simulink model "Chromatic Conveyor"  (R2025a)
settings: Solver=ode3  StartTime=0.0  StopTime=10  RelTol=1e-3  EnableMultiTasking=on
libraries: legoev3lib x4
settings Model: FPTRunName=Active  ExtModeTrigDuration=2  Creator=tstaib  LastModifiedBy=tstaib
settings SolverCC: AlgebraicLoopSolver=TrustRegion  PositivePriorityOrder=on
settings DataIOCC: LimitDataPoints=on  SaveFormat=Array
settings OptimizationCC: ExpressionDepthLimit=2147483647.0  LifeSpan=Inf  MaxStackSize=64
settings DebuggingCC: UnderspecifiedInitializationDetection=Classic  MergeDetectMultiDrivingBlocksExec=none  FcnCallInpInsideContextMsg=warning  UnconnectedInputMsg=warning  UnconnectedOutputMsg=warning  UnconnectedLineMsg=warning  AllowSymbolicDim=off  StateNameClashWarn=warning  SFUnexpectedBacktrackingDiag=warning  SFNoUnconditionalDefaultTransitionDiag=warning  SFExecutionAtInitializationDiag=none  ArithmeticOperatorsInVariantConditions=warning
settings HardwareCC: ProdBitPerPointer=32.0  ProdBitPerSizeT=32.0  ProdBitPerPtrDiffT=32.0  ProdLargestAtomicInteger=Long  ProdWordSize=32.0  ProdHWDeviceType=ARM Compatible->ARM 9  UseEmbeddedCoderFeatures=off
settings ModelReferenceCC: EnableRefExpFcnMdlSchedulingChecks=on  PropagateSignalLabelsOutOfModel=off
settings SFSimCC: SimUseLocalCustomCode=off  CustomCodeUndefinedFunction=UseInterfaceOnly
settings RTWCC: SystemTargetFile=ert.tlc  HardwareBoard=LEGO MINDSTORMS EV3  TemplateMakefile=ert_default_tmf  GenerateReport=on  RTWVerbose=off  RTWUseLocalCustomCode=off  Toolchain=Sourcery G++ Lite v2009q3  BuildConfiguration=Faster Runs  LaunchReport=on  GPUComputeCapability=3.5  Description=Embedded Coder
settings CodeAppCC: ForceParamTrailComments=on  OperatorAnnotations=on  StateflowObjectComments=on  MATLABSourceComments=on
settings ERTTargetCC: ExtModeTransport=0.0  ExtModeStaticAlloc=off  ExtModeMexFile=ext_comm  ExtModeIntrfLevel=Level1  InlinedParameterPlacement=Hierarchical  DynamicArrayContainerType=coder::array  MultiwordLength=2048.0  ERTCustomFileBanners=off  SupportContinuousTime=on  SupportNonInlinedSFcns=on  RemoveResetFunc=off  SupportVariableSizeSignals=on  ModelStepFunctionPrototypeControlCompliant=off
settings ConfigComp: CovMetricSettings=dw  CovSaveCumulativeToWorkspaceVar=on  CovSaveSingleToWorkspaceVar=on  CovExternalEMLEnable=off  CovSFcnEnable=off

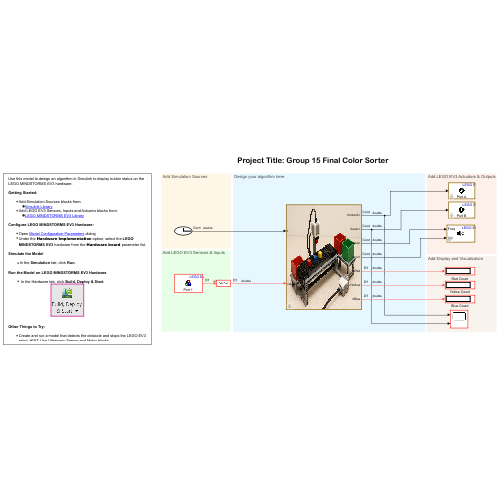
[thumbnail: Simulink's stored preview of the top-level diagram]
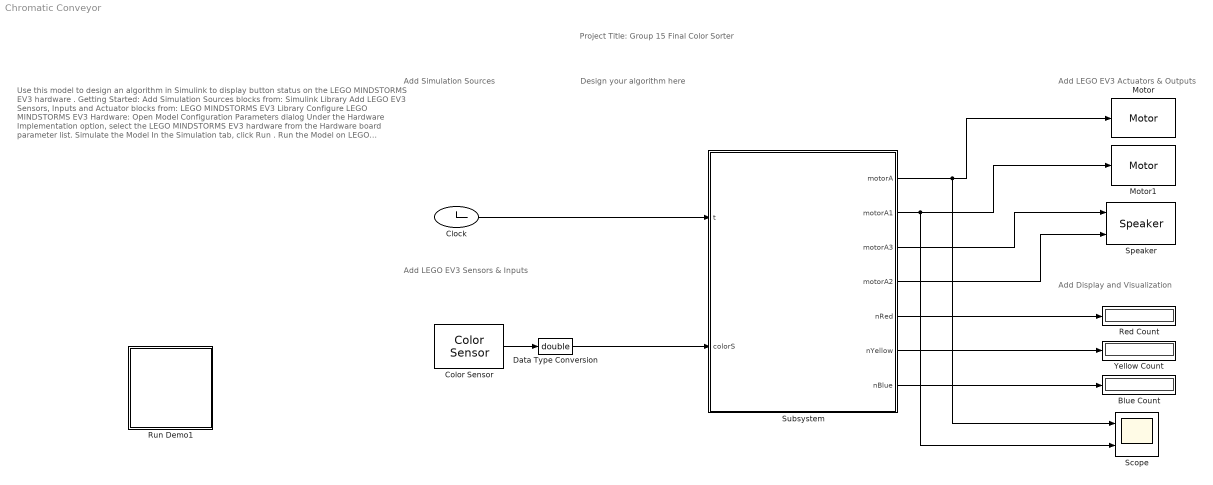
== system Chromatic Conveyor ==
  note: Project Title: Group 15 Final Color Sorter
  note: Add LEGO EV3 Sensors & Inputs
  note: Add LEGO EV3 Actuators & Outputs
  note: Add Display and Visualization
  note: Design your algorithm here
  note: Add Simulation Sources
  note: Use this model to design an algorithm in Simulink to display button status on the LEGO MINDSTORMS EV3 hardware .
      |
      | Getting Started:
      |
      | Add Simulation Sources blocks from:
      | Simulink Library
      | Add LEGO EV3 Sensors, Inputs and Actuator blocks from:
      | LEGO MINDSTORMS EV3 Library
      |
      | Configure LEGO MINDSTORMS EV3 Hardware:
      |
      | Open Model Configuration Parameters dialog
      | Under the Hardware Implementation option, select the LEGO MINDSTORMS EV3 hardware from the Hardware board parameter list.
      |
      | Simulate the Model
      |
      | In the Simulation tab, click Run .
      |
      | Run the Model on LEGO MINDSTORMS EV3 Hardware
      |
      | In the Hardware tab, click Build, Deploy & Start .
      |
      | Other Things to Try:
      |
      | Create and run a model that detects the obstacle and stops the LEGO EV3 robot. HINT: Use Ultrasonic Sensor and Motor blocks.
  Blue Count : Display
  Clock : Clock
  Color Sensor : legoev3lib/Color Sensor  portNumber=1  mode=Reflected light intensity  sampleTime=0.5
  Data Type Conversion : DataTypeConversion  OutDataTypeStr=double  SaturateOnIntegerOverflow=off  RndMeth=Floor
  Motor : legoev3lib/Motor  sportNumber=A  sstopAction=Brake
  Motor1 : legoev3lib/Motor  sportNumber=B  sstopAction=Brake
  Red Count : Display
  Run Demo1 : Subsystem  Description=Controls host-side RTDX processing.
      mask Display: pic=imread('ev3BuildDeployandStart.png');image(pic);
  Scope : Scope  NumInputPorts=2
  Speaker : legoev3lib/Speaker  sinputMode=Frequency and volume  sspeakerFreq=100  sspeakerVolume=50  sspeakerDuration=100
  Subsystem : Subsystem  mask{stopTime=120, speed=30, redR=[70 95], yellowR=[96 100], blueR=[12 20]}
      mask prompts: stopTime "Time On (sec)"; speed "Conveyor Speed"; redR "Red Range [min max]"; yellowR "Yellow Range [min max]"; blueR "Blue Range [min max]"
      mask Display: image('image.png');
  Yellow Count : Display
  wires:
  Clock/1 -> Subsystem/1(t)
  Color Sensor/1 -> Data Type Conversion/1
  Subsystem/1(motorA) -> Scope/1, Motor/1
  Subsystem/2(motorA1) -> Scope/2, Motor1/1
  Data Type Conversion/1 -> Subsystem/2(colorS)
  Subsystem/3(motorA3) -> Speaker/1
  Subsystem/4(motorA2) -> Speaker/2
  Subsystem/5(nRed) -> Red Count/1
  Subsystem/6(nYellow) -> Yellow Count/1
  Subsystem/7(nBlue) -> Blue Count/1

== system Chromatic Conveyor/Run Demo1 ==

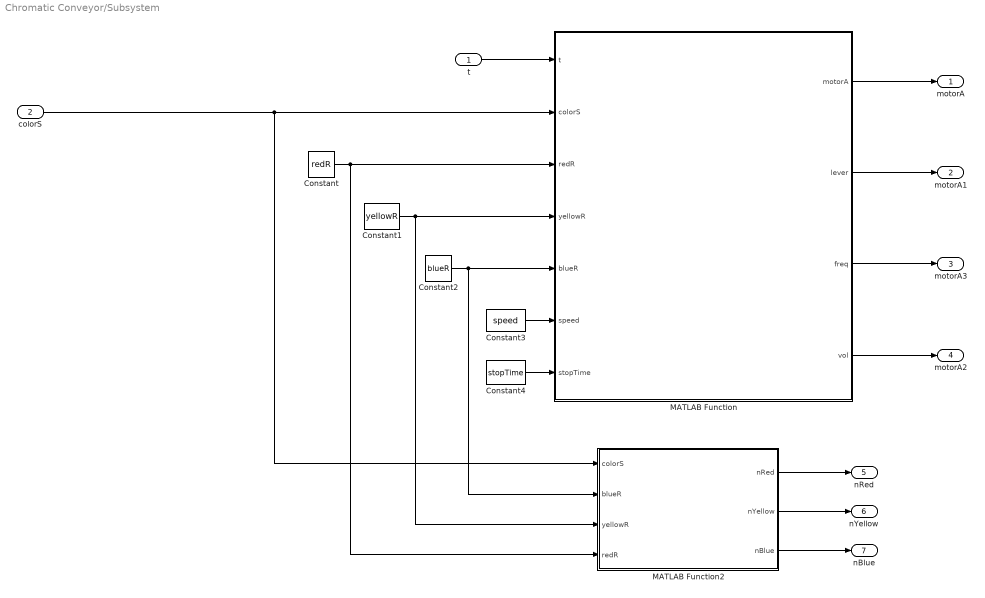
== system Chromatic Conveyor/Subsystem ==
  t : Inport
  colorS : Inport  Port=2
  Constant : Constant  Value=redR
  Constant1 : Constant  Value=yellowR
  Constant2 : Constant  Value=blueR
  Constant3 : Constant  Value=speed
  Constant4 : Constant  Value=stopTime
  MATLAB Function : MATLAB Function  TreatAsAtomicUnit=on
  MATLAB Function2 : MATLAB Function  TreatAsAtomicUnit=on
  motorA : Outport
  motorA1 : Outport  Port=2
  motorA3 : Outport  Port=3
  motorA2 : Outport  Port=4
  nRed : Outport  Port=5
  nYellow : Outport  Port=6
  nBlue : Outport  Port=7
  wires:
  Constant4/1 -> MATLAB Function/7(stopTime)
  Constant3/1 -> MATLAB Function/6(speed)
  Constant2/1 -> MATLAB Function2/2(blueR), MATLAB Function/5(blueR)
  Constant1/1 -> MATLAB Function2/3(yellowR), MATLAB Function/4(yellowR)
  Constant/1 -> MATLAB Function2/4(redR), MATLAB Function/3(redR)
  t/1 -> MATLAB Function/1(t)
  MATLAB Function/1(motorA) -> motorA/1
  MATLAB Function/2(lever) -> motorA1/1
  MATLAB Function/4(vol) -> motorA2/1
  MATLAB Function/3(freq) -> motorA3/1
  MATLAB Function2/1(nRed) -> nRed/1
  MATLAB Function2/2(nYellow) -> nYellow/1
  MATLAB Function2/3(nBlue) -> nBlue/1
  colorS/1 -> MATLAB Function2/1(colorS), MATLAB Function/2(colorS)

== matlab function Chromatic Conveyor/Subsystem/MATLAB Function ==
  data: t input; motorA output; lever output; freq output; colorS input; redR input; yellowR input; blueR input; vol output; speed input; stopTime input
function [motorA, lever, freq, vol] = fcn(t, colorS, redR, yellowR, blueR, speed, stopTime)

% defaults
motorA = 0;
lever  = 0;
vol    = 0;
freq   = 0;

% persistent state for per-brick timing
% state: 0 = idle, 1 = red, 2 = yellow, 3 = blue
persistent state startTime

if isempty(state)
    state     = 0;
    startTime = 0;
end

% 
if t >= stopTime
    state     = 0;     % reset state
    motorA    = 0;
    lever     = 0;
    vol       = 0;
    freq      = 0;
    return;
end

% Conveyor Run time for each brick
runTime = 4;   % seconds


% If we are idle, check the sensor and possibly start a
% new sorting cycle for the current brick.
if state == 0
    if colorS >= redR(1) && colorS <= redR(2)
        state     = 1;      % RED
        startTime = t;
    elseif colorS >= yellowR(1) && colorS <= yellowR(2)
        state     = 2;      % YELLOW
        startTime = t;
    elseif colorS >= blueR(1) && colorS <= blueR(2)
        state     = 3;      % BLUE
        startTime = t;
    end
end


% If we are in an active state, compute how long we've
% been working on this brick and output the appropriate
% motor / lever commands.

elapsed = t - startTime;

switch state
    case 1   % RED 
        if elapsed <= runTime
            motorA = -abs(speed);
            vol    = 10;
            freq   = 400;
        else
            state = 0;
        end

    case 2   % YELLOW
        if elapsed <= runTime
            motorA = +abs(speed);
            vol    = 10;
            freq   = 600;
        else
            state = 0;
        end

    case 3
        if elapsed <= 0.2
            % move lever out, conveyor stopped
            lever  = +10; 
            motorA = 0;
            vol    = 10;
            freq   = 800;

        elseif elapsed <= runTime
            % lever stays out, conveyor runs
            lever  = 0;
            motorA = +abs(speed);

        elseif elapsed <= runTime + 0.5
            % Retract lever
            lever  = -10;
            motorA = 0;

        else
            lever  = 0;
            motorA = 0;
            state  = 0;
        end
    otherwise
end

end

== matlab function Chromatic Conveyor/Subsystem/MATLAB Function2 ==
  data: colorS input; blueR input; yellowR input; nRed output; redR input; nYellow output; nBlue output
function [nRed, nYellow, nBlue] = countColors(colorS, blueR, yellowR, redR)
    % Count how many blocks of each color have passed the sensor
    
    persistent cR cY cB lastClass
    % lastClass: 0 = none, 1 = red, 2 = yellow, 3 = blue
    
    if isempty(cR)
        cR = 0; cY = 0; cB = 0;
        lastClass = 0;
    end
    
    % check range
    isRed    = (colorS >= redR(1))    && (colorS <= redR(2));
    isYellow = (colorS >= yellowR(1)) && (colorS <= yellowR(2));
    isBlue   = (colorS >= blueR(1))   && (colorS <= blueR(2));
    
    currClass = 0;
    if isRed
        currClass = 1;
    elseif isYellow
        currClass = 2;
    elseif isBlue
        currClass = 3;
    end
    
    if currClass ~= 0 && currClass ~= lastClass
        if currClass == 1
            cR = cR + 1;
        elseif currClass == 2
            cY = cY + 1;
        elseif currClass == 3
            cB = cB + 1;
        end
    end
    
    % reset lastClass when no color is detected
    if currClass == 0
        lastClass = 0;
    else
        lastClass = currClass;
    end
    
    % outputs
    nRed    = cR;
    nYellow = cY;
    nBlue   = cB;
end
